simulink model "C_inv_dynamic_sim"  (R2017a)
settings: Solver=ode45  StartTime=0.0  StopTime=10.0  RelTol=1e-3
InitFcn:
  | ImportVars
settings Model: Creator=JayJay  LastModifiedBy=Axel
settings OptimizationCC: LifeSpan=inf
settings DebuggingCC: SFExecutionAtInitializationDiag=none
settings HardwareCC: ProdBitPerSizeT=32  ProdBitPerPtrDiffT=32  ProdWordSize=32  ProdHWDeviceType=Specified

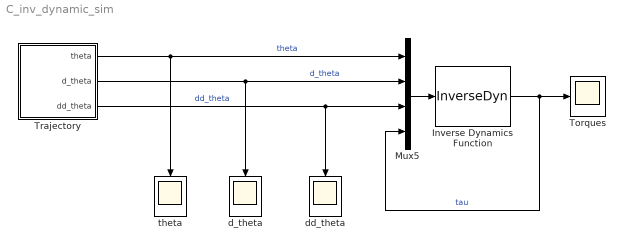
== system C_inv_dynamic_sim ==
  Inverse Dynamics Function : MATLABFcn  MATLABFcn=InverseDyn  OutputDimensions=3
  Mux5 : Mux
  Torques : Scope
  Trajectory : Subsystem
  d_theta : Scope
  dd_theta : Scope
  theta : Scope
  wires:
  Trajectory/2(d_theta) -> Mux5/2, d_theta/1  "d_theta"
  Trajectory/1(theta) -> Mux5/1, theta/1  "theta"
  Mux5/1 -> Inverse Dynamics Function/1
  Inverse Dynamics Function/1 -> Torques/1, Mux5/4  "tau"
  Trajectory/3(dd_theta) -> Mux5/3, dd_theta/1  "dd_theta"

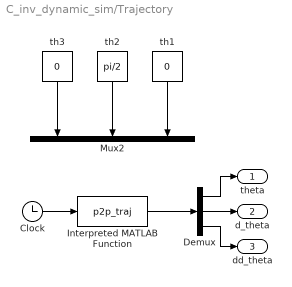
== system C_inv_dynamic_sim/Trajectory ==
  Clock : Clock
  Demux : Demux  Outputs=3
  Interpreted MATLAB Function : MATLABFcn  MATLABFcn=p2p_traj  OutputDimensions=9
  Mux2 : Mux  Inputs=3
  th1 : Constant  Value=0
  th2 : Constant  Value=pi/2
  th3 : Constant  Value=0
  theta : Outport
  d_theta : Outport  Port=2
  dd_theta : Outport  Port=3
  wires:
  Clock/1 -> Interpreted MATLAB Function/1
  Interpreted MATLAB Function/1 -> Demux/1
  Demux/1 -> theta/1
  Demux/2 -> d_theta/1
  Demux/3 -> dd_theta/1
  th3/1 -> Mux2/1
  th1/1 -> Mux2/3
  th2/1 -> Mux2/2
